simulink model "pendulo"  (Simulink 8.7)
settings: Solver=ode14x  StartTime=0.0  StopTime=250  FixedStep=0.1  RelTol=1e-3
settings Model: Creator=Dinis  LastModifiedBy=Dinis
settings SolverCC: ExtrapolationOrder=2
settings DataIOCC: LimitDataPoints=off  SaveFormat=Dataset
settings DebuggingCC: UnderspecifiedInitializationDetection=Simplified  MergeDetectMultiDrivingBlocksExec=error
settings HardwareCC: ProdBitPerPointer=64  ProdLargestAtomicFloat=Float  ProdIntDivRoundTo=Zero  ProdEndianess=LittleEndian  ProdWordSize=64  ProdHWDeviceType=Intel->x86-64 (Windows64)
settings ModelReferenceCC: PropagateSignalLabelsOutOfModel=on
settings ConfigComp: CovModelRefEnable=off

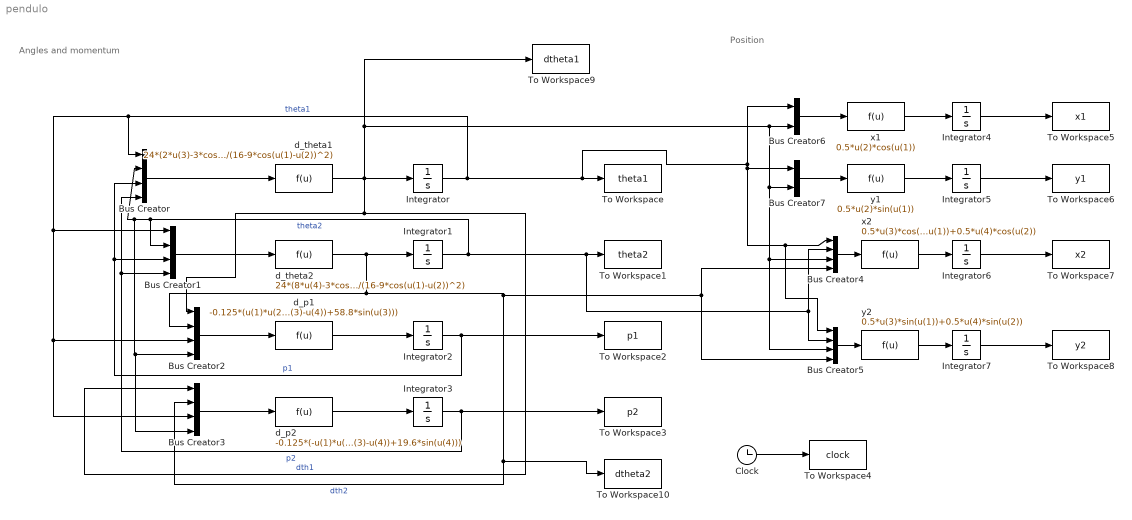
== system pendulo ==
  note: Position
  note: Angles and momentum
  Bus Creator{,1..5} (6 alike) : BusCreator  Inputs=4
  Bus Creator6 : BusCreator  Inputs=2
  Bus Creator7 : BusCreator  Inputs=2
  Clock : Clock
  Integrator : Integrator  InitialCondition=2.2969
  Integrator1 : Integrator  InitialCondition=1.1829
  Integrator2 : Integrator  InitialCondition=-0.014434
  Integrator3 : Integrator  InitialCondition=-0.021817
  Integrator{4..7} (4 alike) : Integrator
  To Workspace : ToWorkspace  VariableName=theta1  SampleTime=-1
  To Workspace1 : ToWorkspace  VariableName=theta2  SampleTime=-1
  To Workspace10 : ToWorkspace  VariableName=dtheta2  SampleTime=-1
  To Workspace2 : ToWorkspace  VariableName=p1  SampleTime=-1
  To Workspace3 : ToWorkspace  VariableName=p2  SampleTime=-1
  To Workspace4 : ToWorkspace  VariableName=clock  SampleTime=-1
  To Workspace5 : ToWorkspace  VariableName=x1  SampleTime=-1
  To Workspace6 : ToWorkspace  VariableName=y1  SampleTime=-1
  To Workspace7 : ToWorkspace  VariableName=x2  SampleTime=-1
  To Workspace8 : ToWorkspace  VariableName=y2  SampleTime=-1
  To Workspace9 : ToWorkspace  VariableName=dtheta1  SampleTime=-1
  d_p1 : Fcn  Expr=-0.125*(u(1)*u(2)*sin(u(3)-u(4))+58.8*sin(u(3)))
  d_p2 : Fcn  Expr=-0.125*(-u(1)*u(2)*sin(u(3)-u(4))+19.6*sin(u(4)))
  d_theta1 : Fcn  Expr=24*(2*u(3)-3*cos(u(1)-u(2))*u(4))/(16-9*cos(u(1)-u(2))^2)
  d_theta2 : Fcn  Expr=24*(8*u(4)-3*cos(u(1)-u(2))*u(3))/(16-9*cos(u(1)-u(2))^2)
  x1 : Fcn  Expr=0.5*u(2)*cos(u(1))
  x2 : Fcn  Expr=0.5*u(3)*cos(u(1))+0.5*u(4)*cos(u(2))
  y1 : Fcn  Expr=0.5*u(2)*sin(u(1))
  y2 : Fcn  Expr=0.5*u(3)*sin(u(1))+0.5*u(4)*sin(u(2))
  wires:
  d_p1/1 -> Integrator2/1
  d_p2/1 -> Integrator3/1
  Integrator1/1 -> Bus Creator4/2, Bus Creator5/2, To Workspace1/1, Bus Creator1/2, Bus Creator3/4, Bus Creator2/4, Bus Creator/2  "theta2"
  Integrator2/1 -> To Workspace2/1, Bus Creator1/3, Bus Creator/3  "p1"
  Integrator3/1 -> To Workspace3/1, Bus Creator1/4, Bus Creator/4  "p2"
  Integrator/1 -> Bus Creator6/1, Bus Creator7/1, Bus Creator5/1, Bus Creator4/1, To Workspace/1, Bus Creator/1, Bus Creator3/3, Bus Creator2/3, Bus Creator1/1  "theta1"
  d_theta1/1 -> To Workspace9/1, Bus Creator5/3, Bus Creator4/3, Bus Creator7/2, Bus Creator6/2, Bus Creator3/1, Bus Creator2/1, Integrator/1  "dth1"
  d_theta2/1 -> Bus Creator5/4, Bus Creator4/4, To Workspace10/1, Bus Creator3/2, Bus Creator2/2, Integrator1/1  "dth2"
  Clock/1 -> To Workspace4/1
  Bus Creator5/1 -> y2/1
  Bus Creator4/1 -> x2/1
  Bus Creator2/1 -> d_p1/1
  Bus Creator3/1 -> d_p2/1
  Bus Creator1/1 -> d_theta2/1
  Bus Creator/1 -> d_theta1/1
  x1/1 -> Integrator4/1
  Integrator4/1 -> To Workspace5/1
  y1/1 -> Integrator5/1
  Integrator5/1 -> To Workspace6/1
  x2/1 -> Integrator6/1
  Integrator6/1 -> To Workspace7/1
  y2/1 -> Integrator7/1
  Integrator7/1 -> To Workspace8/1
  Bus Creator6/1 -> x1/1
  Bus Creator7/1 -> y1/1
